simulink model "frameBasedStatistics"  (R2024a)
settings: Solver=FixedStepDiscrete  StartTime=0.0  StopTime=1  RelTol=1e-3
libraries: visionsources x1
Description:
  | Sobel Edge Detection Using the MATLAB(R) Function Block
  | This example shows how to use HDL Coder(TM) to check,
  | generate, and verify HDL code for a Sobel Edge Detection
  | block built using the MATLAB Function block.
settings Model: FPTRunName=Active  Creator=The MathWorks, Inc.  LastModifiedBy=dskap
settings SolverCC: AlgebraicLoopSolver=TrustRegion
settings DataIOCC: LimitDataPoints=on  SaveFormat=Array  SignalLogging=off  ReturnWorkspaceOutputs=off
settings OptimizationCC: BlockReduction=off  ConditionallyExecuteInputs=off  DefaultParameterBehavior=Inlined  ExpressionDepthLimit=2147483647  InitFltsAndDblsToZero=on  EfficientMapNaN2IntZero=off  LifeSpan=inf
settings DebuggingCC: AlgebraicLoopMsg=error  SaveWithParameterizedLinksMsg=none  UnderspecifiedInitializationDetection=Classic  MergeDetectMultiDrivingBlocksExec=none  SignalResolutionControl=TryResolveAllWithWarning  MultiTaskDSMMsg=warning  MultiTaskCondExecSysMsg=none  SingleTaskRateTransMsg=error  IntegerOverflowMsg=none  ParameterPrecisionLossMsg=none  FcnCallInpInsideContextMsg=warning  UnconnectedInputMsg=warning  UnconnectedOutputMsg=warning  UnconnectedLineMsg=warning  AllowSymbolicDim=off  StateNameClashWarn=warning  StrictBusMsg=ErrorOnBusTreatedAsVector  SFUnexpectedBacktrackingDiag=warning  SFNoUnconditionalDefaultTransitionDiag=warning  SFExecutionAtInitializationDiag=none  IntegerSaturationMsg=none  ArithmeticOperatorsInVariantConditions=warning
settings HardwareCC: ProdBitPerPointer=32  ProdBitPerSizeT=32  ProdBitPerPtrDiffT=32  ProdLargestAtomicFloat=None  ProdIntDivRoundTo=Undefined  ProdEndianess=Unspecified  ProdWordSize=32  ProdHWDeviceType=ASIC/FPGA  TargetHWDeviceType=32-bit Generic  ProdEqTarget=off
settings ModelReferenceCC: EnableRefExpFcnMdlSchedulingChecks=on  PropagateSignalLabelsOutOfModel=off
settings SFSimCC: SimUseLocalCustomCode=off  CustomCodeUndefinedFunction=UseInterfaceOnly
settings RTWCC: RTWUseLocalCustomCode=off  GPUComputeCapability=3.5  DLArmComputeVersion=19.05
settings CodeAppCC: StateflowObjectComments=on
settings GRTTargetCC: TargetFcnLib=ansi_tfl_tmw.mat  TargetLangStandard=C89/C90 (ANSI)  CombineOutputUpdateFcns=off  GRTInterface=on
settings ConfigComp: CovMetricSettings=dw  CovSaveCumulativeToWorkspaceVar=on  CovSaveSingleToWorkspaceVar=on  CovExternalEMLEnable=off

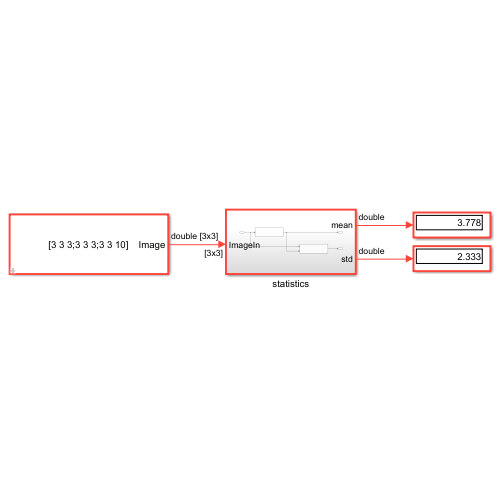
[thumbnail: Simulink's stored preview of the top-level diagram]
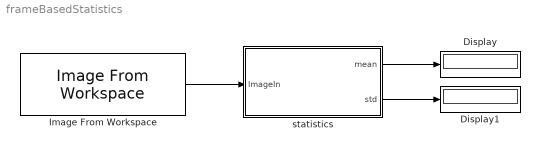
== system frameBasedStatistics ==
  Display : Display
  Display1 : Display
  Image From Workspace : visionsources/Image From Workspace  Tag=vipblks_nd  ImageValue=[3 3 3;3 3 3;3 3 10]  Ts=1  imagePorts=One multidimensional signal  OutPortLabels=R|G|B  ImageDataType=Inherit from 'Value'  Signed=on  WordLength=16  sdImageDataType=sfix(16)  FractionLengthMode=User-defined  FractionLength=15
  statistics : Subsystem
  wires:
  Image From Workspace/1 -> statistics/1(ImageIn)
  statistics/1(mean) -> Display/1
  statistics/2(std) -> Display1/1

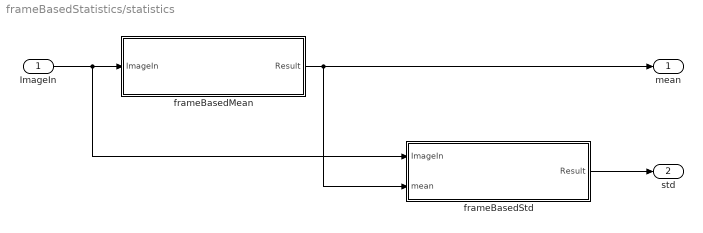
== system frameBasedStatistics/statistics ==
  ImageIn : Inport
  frameBasedMean : MATLAB Function  TreatAsAtomicUnit=on
  frameBasedStd : MATLAB Function  TreatAsAtomicUnit=on
  mean : Outport
  std : Outport  Port=2
  wires:
  frameBasedStd/1(Result) -> std/1
  ImageIn/1 -> frameBasedStd/1(ImageIn), frameBasedMean/1(ImageIn)
  frameBasedMean/1(Result) -> frameBasedStd/2(mean), mean/1

== matlab function frameBasedStatistics/statistics/frameBasedStd ==
  data: Result output; ImageIn input; mean input
function Result   = frameBasedStd(ImageIn, mean)
    accumulator2 = 0;
    Result = hdl.iteratorfun(@max_fun2, ImageIn, accumulator2,mean); 
end
 
function accumulator2 = max_fun2(sample, accumulator2, idx, mean)
  temp = (sample-mean)^2;
  accumulator2 = accumulator2 + temp;
  
  if idx == 9
    accumulator2 = (accumulator2/8)^.5;
  end
end

== matlab function frameBasedStatistics/statistics/frameBasedMean ==
  data: Result output; ImageIn input
function Result   = frameBasedMean(ImageIn)
    accumulator = 0;    
    % pull image size and pass into iterator
    Result = hdl.iteratorfun(@max_fun, ImageIn, accumulator);
end
 
function accumulator = max_fun(sample, accumulator, idx)
  accumulator = accumulator + sample;
  if idx == 9
    accumulator = accumulator / 9;
  end
end
